simulink library "Tracked_Surface"  (Simulink 8.2)
settings: Solver=ode45  StartTime=0.0  StopTime=10.0  RelTol=1e-3
settings Model: Creator=lena.frank  LastModifiedBy=drhf

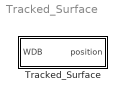
== system Tracked_Surface ==
  Tracked_Surface : Subsystem  mask(tracked surface){tracktype=two axis tracking, inc=0, azi=0, rot=0, time=0}
      mask prompts: tracktype "tracking type"; inc "inclination of surface or axis [degrees]"; azi "azimuth of surface or axis (0° = south, -90° = east) [degree]"; rot "rotation of surface or axis [degree]"; time "tracking time [s]"
      mask help: Performs a collector tracking around a given axis. You may specify the time in seconds between two trackings.
      mask Help: web(fullfile(path_carnot('help'),'Tracked_Surface.html'),'-helpbrowser')
      mask TypeOptions tracktype: axis is collector riser | vertical axis | two axis tracking | fixed surface

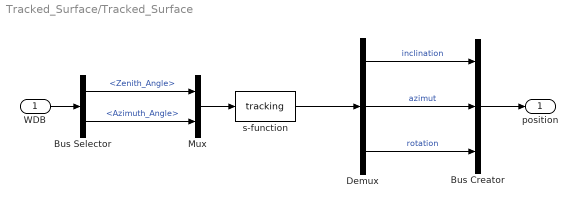
== system Tracked_Surface/Tracked_Surface ==
  WDB : Inport
  Bus Creator : BusCreator  Inputs=3
  Bus Selector : BusSelector  OutputSignals=Zenith_Angle,Azimuth_Angle
  Demux : Demux  Outputs=3
  Mux : Mux  Inputs=2
  s-function : S-Function  FunctionName=tracking  Parameters=tracktype time inc azi rot  EnableBusSupport=off
  position : Outport
  wires:
  Bus Creator/1 -> position/1
  s-function/1 -> Demux/1
  Demux/3 -> Bus Creator/3  "rotation"
  Demux/2 -> Bus Creator/2  "azimut"
  Demux/1 -> Bus Creator/1  "inclination"
  WDB/1 -> Bus Selector/1
  Mux/1 -> s-function/1
  Bus Selector/1 -> Mux/1  "<Zenith_Angle>"
  Bus Selector/2 -> Mux/2  "<Azimuth_Angle>"
